simulink model "Lya_nonlinear_2016a"  (R2016a)
settings: Solver=FixedStepAuto  SolverMode=SingleTasking  StartTime=0.0  StopTime=10.0  FixedStep=0.001  RelTol=1e-3
values from neighbouring files (symbols this model uses):
  alpha0 = 0    [Para.m]
  F1 = 2*wc    (= 20)    [Para.m]
  F2 = wc^2    (= 100)    [Para.m]
  Kd = 100    [Para.m]
  Ki = 100    [Para.m]
  Kp = 100    [Para.m]
  namuta = 50    [Para.m]
settings Model: Creator=chengqian  LastModifiedBy=chengqian
settings DebuggingCC: SFUnexpectedBacktrackingDiag=error  SFNoUnconditionalDefaultTransitionDiag=error
settings SFSimCC: SimUseLocalCustomCode=on
settings RTWCC: RTWUseLocalCustomCode=on
settings GRTTargetCC: TargetLangStandard=C99 (ISO)  GeneratePreprocessorConditionals=Use local settings
settings ConfigComp: CovMetricSettings=dwe  CovHtmlReporting=off  CovSaveCumulativeToWorkspaceVar=off  CovSaveSingleToWorkspaceVar=off  CovExternalEMLEnable=on

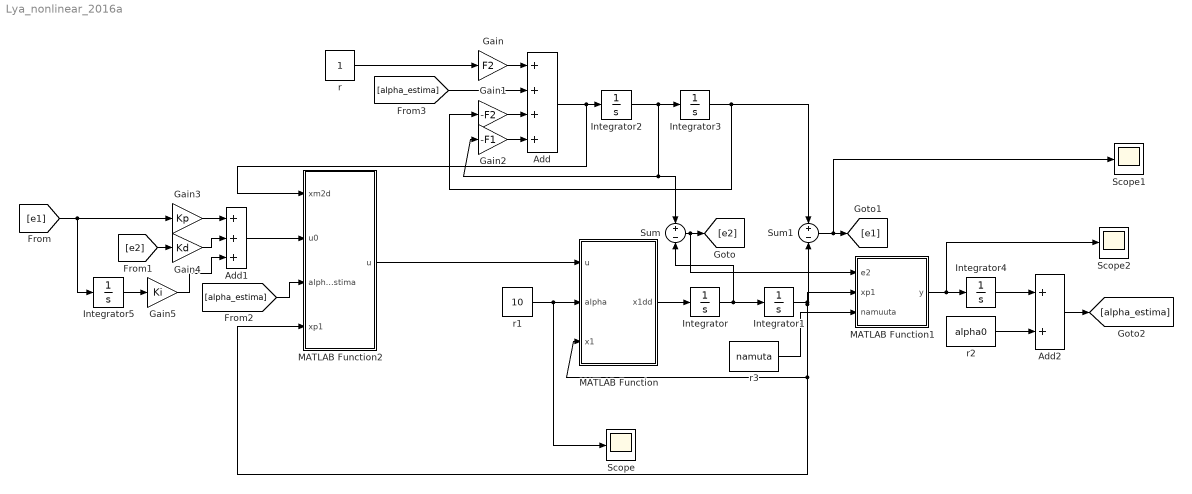
== system Lya_nonlinear_2016a ==
  Add : Sum  Inputs=++++
  Add1 : Sum  Inputs=+++
  Add2 : Sum
  Gain : Gain  Gain=F2
  Gain1 : Gain  Gain=-F2
  Gain2 : Gain  Gain=-F1
  Gain3 : Gain  Gain=Kp
  Gain4 : Gain  Gain=Kd
  Gain5 : Gain  Gain=Ki
  Integrator{,1..5} (6 alike) : Integrator
  MATLAB Function : MATLAB Function  TreatAsAtomicUnit=on
  MATLAB Function1 : MATLAB Function  TreatAsAtomicUnit=on
  MATLAB Function2 : MATLAB Function  TreatAsAtomicUnit=on
  Scope : Scope
  Scope1 : Scope
  Scope2 : Scope
  Sum : Sum  Inputs=+|-
  Sum1 : Sum  Inputs=+|-
  r : Constant
  r1 : Constant  Value=10
  r2 : Constant  Value=alpha0
  r3 : Constant  Value=namuta
  wires:
  MATLAB Function/1(x1dd) -> Integrator/1
  Integrator/1 -> Integrator1/1, Sum/2
  Integrator1/1 -> Sum1/2, MATLAB Function2/4(xp1), MATLAB Function/3(x1), MATLAB Function1/2(xp1)
  r1/1 -> MATLAB Function/2(alpha), Scope/1
  Gain/1 -> Add/1
  Add/1 -> MATLAB Function2/1(xm2d), Integrator2/1
  Gain1/1 -> Add/3
  Integrator2/1 -> Sum/1, Gain2/1, Integrator3/1
  Integrator3/1 -> Sum1/1, Gain1/1
  Gain2/1 -> Add/4
  r/1 -> Gain/1
  MATLAB Function2/1(u) -> MATLAB Function/1(u)
  Sum/1 -> MATLAB Function1/1(e2), [e2]
  Sum1/1 -> Scope1/1, [e1]
  Add1/1 -> MATLAB Function2/2(u0)
  Gain3/1 -> Add1/1
  [e1] -> Integrator5/1, Gain3/1
  [e2] -> Gain4/1
  Gain4/1 -> Add1/2
  MATLAB Function1/1(y) -> Scope2/1, Integrator4/1
  Integrator4/1 -> Add2/1
  r2/1 -> Add2/2
  Add2/1 -> [alpha_estima]
  [alpha_estima] -> MATLAB Function2/3(alpha_estima)
  [alpha_estima] -> Add/2
  r3/1 -> MATLAB Function1/3(namuuta)
  Integrator5/1 -> Gain5/1
  Gain5/1 -> Add1/3

== matlab function Lya_nonlinear_2016a/MATLAB Function1 ==
  data: e2 input; y output; xp1 input; namuuta input
function y = fcn(e2,xp1,namuuta)

y = -xp1^3*e2/namuuta;

== matlab function Lya_nonlinear_2016a/MATLAB Function ==
  data: u input; x1dd output; alpha input; x1 input
function x1dd = fcn(u,alpha,x1)

m=1;

x1dd = -alpha*x1^3/m + u/m;

== matlab function Lya_nonlinear_2016a/MATLAB Function2 ==
  data: xm2d input; u0 input; u output; alpha_estima input; xp1 input
function u = fcn(xm2d,u0,alpha_estima,xp1)
m=1;
u = m*(u0+xm2d+alpha_estima*xp1^3/m);
